simulink model "ControlDC_Velocidad_RTWT_6014_2016_Pololu"  (R2016a)
settings: Solver=ode5  StartTime=0.0  StopTime=inf  FixedStep=T  RelTol=1e-3
undefined symbols (not defined in the file or in its folder): National_Instruments, PCI, T
libraries: sldrtlib x3, simulink_need_slupdate x1
settings Model: SimulationMode=external  Creator=Rafa  LastModifiedBy=Docencia
settings DataIOCC: LimitDataPoints=on  SaveFormat=Array  SignalLoggingSaveFormat=ModelDataLogs
settings OptimizationCC: ExpressionDepthLimit=2147483647
settings DebuggingCC: UnderspecifiedInitializationDetection=Classic  MergeDetectMultiDrivingBlocksExec=none  SolverPrmCheckMsg=warning  FcnCallInpInsideContextMsg=UseLocalSettings  StateNameClashWarn=warning
settings HardwareCC: ProdBitPerLong=64  ProdLargestAtomicFloat=None  ProdHWDeviceType=Intel->x86-64  TargetBitPerLong=64  TargetBitPerPointer=64  TargetIntDivRoundTo=Zero  TargetEndianess=LittleEndian  TargetWordSize=64  TargetHWDeviceType=Intel->x86-64
settings ModelReferenceCC: PropagateSignalLabelsOutOfModel=off
settings RTWCC: SystemTargetFile=sldrt.tlc  TemplateMakefile=sldrt.tmf  Description=Simulink Desktop Real-Time  RTWCompilerOptimization=on
settings CodeAppCC: MaxIdLength=95
settings SimulinkDesktopRealTimeCC: TargetPreCompLibLocation=C:\Program Files\MATLAB\R2016a\toolbox\sldrt\lib\win64  TargetLangStandard=C89/C90 (ANSI)  SupportVariableSizeSignals=off
settings ConfigComp: CovModelRefEnable=Off

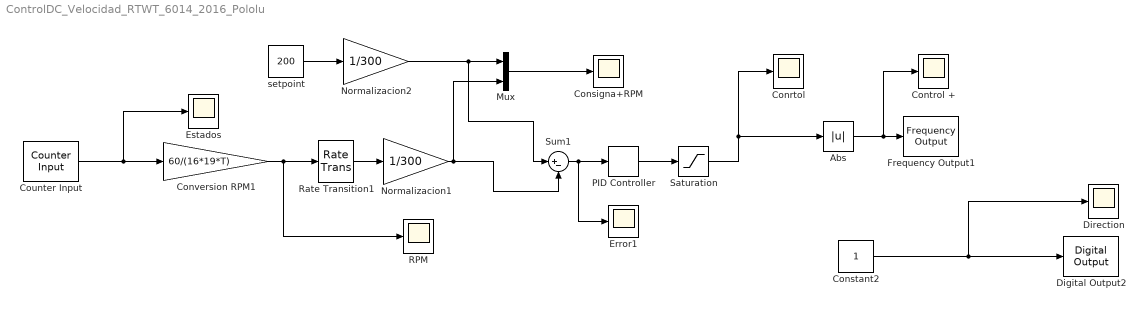
== system ControlDC_Velocidad_RTWT_6014_2016_Pololu ==
  Abs : Abs
  Conrtol : Scope
  Consigna+RPM : Scope
  Constant2 : Constant
  Control + : Scope
  Conversion RPM1 : Gain  Gain=60/(16*19*T)
  Counter Input : sldrtlib/Counter Input  SampleTime=T  MaxMissedTicks=10  ShowMissedTicks=off  YieldWhenWaiting=off  DrvName=National_Instruments/PCI-6014  DrvAddress=4294967295  DrvOptions=[1 0 1 0 1 1]  Channels=2  ResetMode=2  CounterEdge=2  CounterGate=1  DataType=1
      settings: AttributesFormatString=National Instruments\nPCI-6014 [auto]
  Digital Output2 : sldrtlib/Digital Output  SampleTime=T  MaxMissedTicks=10  ShowMissedTicks=off  YieldWhenWaiting=off  DrvName=National_Instruments/PCI-6014  DrvAddress=4294967295  DrvOptions=[1 0 1 0 1 1]  Channels=1  BitMode=1  InitialValue=0  FinalValue=0
      settings: AttributesFormatString=National Instruments\nPCI-6014 [auto]
  Direction : Scope
  Error1 : Scope
  Estados : Scope
  Frequency Output1 : sldrtlib/Frequency Output  SampleTime=T  MaxMissedTicks=10  ShowMissedTicks=off  YieldWhenWaiting=off  DrvName=National_Instruments/PCI-6014  DrvAddress=4294967295  DrvOptions=[1 0 1 0 1 1]  Channels=1  FrequencySource=1  Frequency=200  FrequencyFinalValue=[]  DutySource=2  Duty=0  DutyFinalValue=0
      settings: AttributesFormatString=National Instruments\nPCI-6014 [auto]
  Mux : Mux  Inputs=2
  Normalizacion1 : Gain  Gain=1/300
  Normalizacion2 : Gain  Gain=1/300
  PID Controller : simulink_need_slupdate/PID Controller  P=0.4  I=0.5  D=0
  RPM : Scope
  Rate Transition1 : RateTransition  OutPortSampleTime=T
  Saturation : Saturate  UpperLimit=1  LowerLimit=-1
  Sum1 : Sum  Inputs=|+-
  setpoint : Constant  Value=200
  wires:
  Abs/1 -> Frequency Output1/1, Control +/1
  setpoint/1 -> Normalizacion2/1
  Sum1/1 -> PID Controller/1, Error1/1
  Normalizacion2/1 -> Mux/1, Sum1/1
  PID Controller/1 -> Saturation/1
  Mux/1 -> Consigna+RPM/1
  Counter Input/1 -> Conversion RPM1/1, Estados/1
  Conversion RPM1/1 -> Rate Transition1/1, RPM/1
  Normalizacion1/1 -> Mux/2, Sum1/2
  Rate Transition1/1 -> Normalizacion1/1
  Saturation/1 -> Abs/1, Conrtol/1
  Constant2/1 -> Digital Output2/1, Direction/1
